simulink model "BCM_C1A_CombiSwitch_9"  (R2018b)
settings: Solver=FixedStepDiscrete  StartTime=0.0  StopTime=10.0  FixedStep=0.01  RelTol=1e-3
undefined symbols (not defined in the file or in its folder): TYP_CSW_INT_POSITION, TYP_EXT_LIGHTS, TYP_FRONT_WIPER, TYP_LIGHTING_CSW, TYP_REAR_WIPER, TYP_VEHICLE_STATE
libraries: Renault_Library x80, library_BCM x2
(part 1 of 3)
settings Model: Creator=a205328  LastModifiedBy=40005501
settings DataIOCC: LimitDataPoints=on  SaveFormat=StructureWithTime  SignalLoggingSaveFormat=ModelDataLogs
settings OptimizationCC: ExpressionDepthLimit=2147483647  LifeSpan=inf
settings DebuggingCC: UnderspecifiedInitializationDetection=Classic  MergeDetectMultiDrivingBlocksExec=none  SolverPrmCheckMsg=warning  InheritedTsInSrcMsg=none  FcnCallInpInsideContextMsg=warning  StateNameClashWarn=warning  SFUnexpectedBacktrackingDiag=warning  SFNoUnconditionalDefaultTransitionDiag=warning  SFExecutionAtInitializationDiag=none
settings HardwareCC: ProdBitPerPointer=32  ProdBitPerSizeT=32  ProdBitPerPtrDiffT=32  ProdLargestAtomicFloat=None  ProdIntDivRoundTo=Undefined  ProdEndianess=Unspecified  ProdWordSize=32  ProdHWDeviceType=32-bit Generic  TargetBitPerPointer=64  TargetBitPerSizeT=64  TargetBitPerPtrDiffT=64  TargetLongLongMode=on  TargetIntDivRoundTo=Zero  TargetEndianess=LittleEndian  TargetWordSize=64  TargetHWDeviceType=MATLAB Host  ProdEqTarget=off
settings ModelReferenceCC: PropagateSignalLabelsOutOfModel=off
settings SFSimCC: SimUseLocalCustomCode=off
settings RTWCC: Description=Generic Real-Time Target  RTWUseLocalCustomCode=off
settings CodeAppCC: StateflowObjectComments=on
settings GRTTargetCC: TargetLangStandard=C89/C90 (ANSI)  GeneratePreprocessorConditionals=Disable all  CombineOutputUpdateFcns=off  MatFileLogging=off  SupportNonFinite=off  GRTInterface=on
settings ConfigComp: CovMetricSettings=dcmw  CovHTMLOptions=-sRT=1 -aTS=1 -bRG=1 -bTC=1 -hTR=0 -nFC=0 -scm=1 -bcm=1 -xEv=0  CovHtmlReporting=on  CovSaveCumulativeToWorkspaceVar=on  CovSaveSingleToWorkspaceVar=on  CovExternalEMLEnable=off  DVMaxTestCaseSteps=500  DVTestSuiteOptimization=CombinedObjectives (Nonlinear Extended)  DVDetectDeadLogic=on  DVDetectActiveLogic=on  DVDetectDivisionByZero=off  DVDetectIntegerOverflow=off  DVSaveReport=on

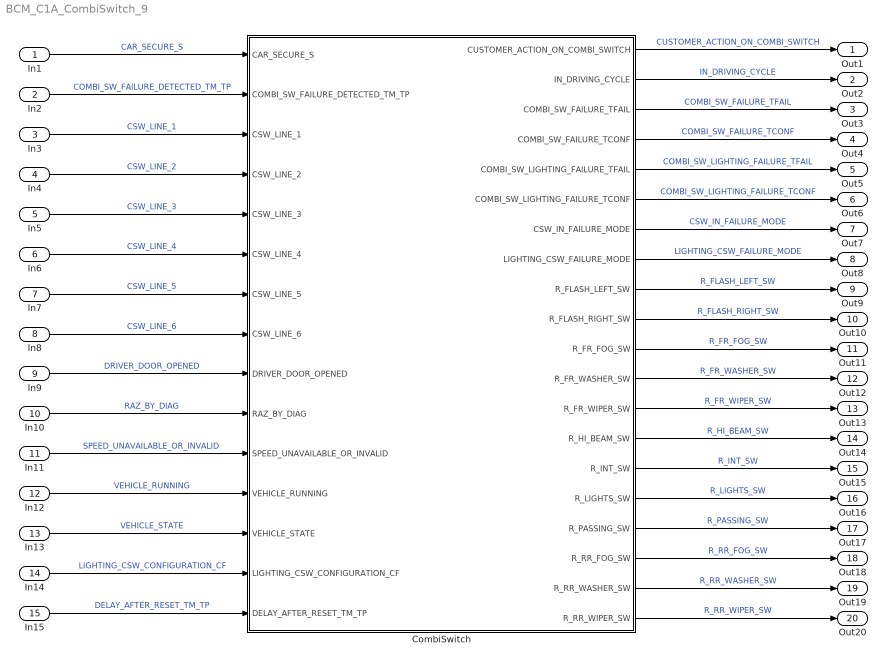
== system BCM_C1A_CombiSwitch_9 ==
  In1 : Inport
  In2 : Inport  Port=2
  In3 : Inport  Port=3
  In4 : Inport  Port=4
  In5 : Inport  Port=5
  In6 : Inport  Port=6
  In7 : Inport  Port=7
  In8 : Inport  Port=8
  In9 : Inport  Port=9
  In10 : Inport  Port=10
  In11 : Inport  Port=11
  In12 : Inport  Port=12
  In13 : Inport  Port=13
  In14 : Inport  Port=14
  In15 : Inport  Port=15
  CombiSwitch : Subsystem  Tag=[RUNNABLE]
  Out1 : Outport
  Out2 : Outport  Port=2
  Out3 : Outport  Port=3
  Out4 : Outport  Port=4
  Out5 : Outport  Port=5
  Out6 : Outport  Port=6
  Out7 : Outport  Port=7
  Out8 : Outport  Port=8
  Out9 : Outport  Port=9
  Out10 : Outport  Port=10
  Out11 : Outport  Port=11
  Out12 : Outport  Port=12
  Out13 : Outport  Port=13
  Out14 : Outport  Port=14
  Out15 : Outport  Port=15
  Out16 : Outport  Port=16
  Out17 : Outport  Port=17
  Out18 : Outport  Port=18
  Out19 : Outport  Port=19
  Out20 : Outport  Port=20
  wires:
  In1/1 -> CombiSwitch/1(CAR_SECURE_S)  "CAR_SECURE_S"
  In2/1 -> CombiSwitch/2(COMBI_SW_FAILURE_DETECTED_TM_TP)  "COMBI_SW_FAILURE_DETECTED_TM_TP"
  In3/1 -> CombiSwitch/3(CSW_LINE_1)  "CSW_LINE_1"
  In4/1 -> CombiSwitch/4(CSW_LINE_2)  "CSW_LINE_2"
  In5/1 -> CombiSwitch/5(CSW_LINE_3)  "CSW_LINE_3"
  In6/1 -> CombiSwitch/6(CSW_LINE_4)  "CSW_LINE_4"
  In7/1 -> CombiSwitch/7(CSW_LINE_5)  "CSW_LINE_5"
  In8/1 -> CombiSwitch/8(CSW_LINE_6)  "CSW_LINE_6"
  In9/1 -> CombiSwitch/9(DRIVER_DOOR_OPENED)  "DRIVER_DOOR_OPENED"
  In10/1 -> CombiSwitch/10(RAZ_BY_DIAG)  "RAZ_BY_DIAG"
  In11/1 -> CombiSwitch/11(SPEED_UNAVAILABLE_OR_INVALID)  "SPEED_UNAVAILABLE_OR_INVALID"
  In12/1 -> CombiSwitch/12(VEHICLE_RUNNING)  "VEHICLE_RUNNING"
  In13/1 -> CombiSwitch/13(VEHICLE_STATE)  "VEHICLE_STATE"
  In14/1 -> CombiSwitch/14(LIGHTING_CSW_CONFIGURATION_CF)  "LIGHTING_CSW_CONFIGURATION_CF"
  In15/1 -> CombiSwitch/15(DELAY_AFTER_RESET_TM_TP)  "DELAY_AFTER_RESET_TM_TP"
  CombiSwitch/1(CUSTOMER_ACTION_ON_COMBI_SWITCH) -> Out1/1  "CUSTOMER_ACTION_ON_COMBI_SWITCH"
  CombiSwitch/2(IN_DRIVING_CYCLE) -> Out2/1  "IN_DRIVING_CYCLE"
  CombiSwitch/3(COMBI_SW_FAILURE_TFAIL) -> Out3/1  "COMBI_SW_FAILURE_TFAIL"
  CombiSwitch/4(COMBI_SW_FAILURE_TCONF) -> Out4/1  "COMBI_SW_FAILURE_TCONF"
  CombiSwitch/5(COMBI_SW_LIGHTING_FAILURE_TFAIL) -> Out5/1  "COMBI_SW_LIGHTING_FAILURE_TFAIL"
  CombiSwitch/6(COMBI_SW_LIGHTING_FAILURE_TCONF) -> Out6/1  "COMBI_SW_LIGHTING_FAILURE_TCONF"
  CombiSwitch/7(CSW_IN_FAILURE_MODE) -> Out7/1  "CSW_IN_FAILURE_MODE"
  CombiSwitch/8(LIGHTING_CSW_FAILURE_MODE) -> Out8/1  "LIGHTING_CSW_FAILURE_MODE"
  CombiSwitch/9(R_FLASH_LEFT_SW) -> Out9/1  "R_FLASH_LEFT_SW"
  CombiSwitch/10(R_FLASH_RIGHT_SW) -> Out10/1  "R_FLASH_RIGHT_SW"
  CombiSwitch/11(R_FR_FOG_SW) -> Out11/1  "R_FR_FOG_SW"
  CombiSwitch/12(R_FR_WASHER_SW) -> Out12/1  "R_FR_WASHER_SW"
  CombiSwitch/13(R_FR_WIPER_SW) -> Out13/1  "R_FR_WIPER_SW"
  CombiSwitch/14(R_HI_BEAM_SW) -> Out14/1  "R_HI_BEAM_SW"
  CombiSwitch/15(R_INT_SW) -> Out15/1  "R_INT_SW"
  CombiSwitch/16(R_LIGHTS_SW) -> Out16/1  "R_LIGHTS_SW"
  CombiSwitch/17(R_PASSING_SW) -> Out17/1  "R_PASSING_SW"
  CombiSwitch/18(R_RR_FOG_SW) -> Out18/1  "R_RR_FOG_SW"
  CombiSwitch/19(R_RR_WASHER_SW) -> Out19/1  "R_RR_WASHER_SW"
  CombiSwitch/20(R_RR_WIPER_SW) -> Out20/1  "R_RR_WIPER_SW"

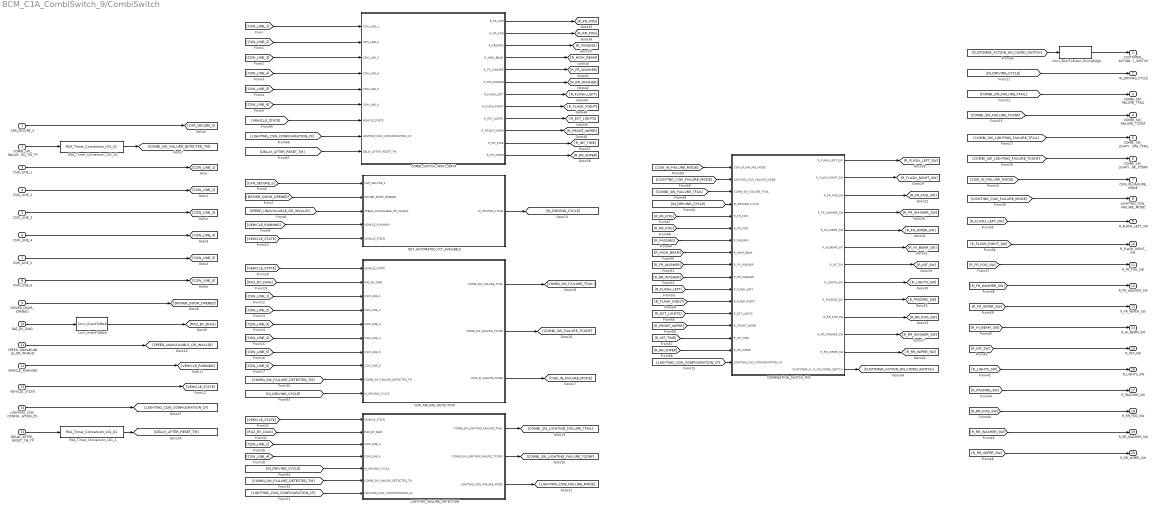
== system BCM_C1A_CombiSwitch_9/CombiSwitch ==
  CAR_SECURE_S : Inport  OutDataTypeStr=boolean
      settings: AttributesFormatString=Type : %<OutDataTypeStr>
  COMBI_SW_FAILURE_DETECTED_TM_TP : Inport  Port=2  OutDataTypeStr=uint16
      settings: AttributesFormatString=Type : %<OutDataTypeStr>
  CSW_LINE_1 : Inport  Port=3  OutDataTypeStr=boolean  PortDimensions=6
      settings: AttributesFormatString=Type : %<OutDataTypeStr>
  CSW_LINE_2 : Inport  Port=4  OutDataTypeStr=boolean  PortDimensions=6
      settings: AttributesFormatString=Type : %<OutDataTypeStr>
  CSW_LINE_3 : Inport  Port=5  OutDataTypeStr=boolean  PortDimensions=6
      settings: AttributesFormatString=Type : %<OutDataTypeStr>
  CSW_LINE_4 : Inport  Port=6  OutDataTypeStr=boolean  PortDimensions=6
      settings: AttributesFormatString=Type : %<OutDataTypeStr>
  CSW_LINE_5 : Inport  Port=7  OutDataTypeStr=boolean  PortDimensions=6
      settings: AttributesFormatString=Type : %<OutDataTypeStr>
  CSW_LINE_6 : Inport  Port=8  OutDataTypeStr=boolean  PortDimensions=6
      settings: AttributesFormatString=Type : %<OutDataTypeStr>
  DRIVER_DOOR_OPENED : Inport  Port=9  OutDataTypeStr=boolean
      settings: AttributesFormatString=Type : %<OutDataTypeStr>
  RAZ_BY_DIAG : Inport  Port=10  OutDataTypeStr=Enum: TYP_EVENT
      settings: AttributesFormatString=Type : %<OutDataTypeStr>
  SPEED_UNAVAILABLE_OR_INVALID : Inport  Port=11  OutDataTypeStr=boolean
      settings: AttributesFormatString=Type : %<OutDataTypeStr>
  VEHICLE_RUNNING : Inport  Port=12  OutDataTypeStr=boolean
      settings: AttributesFormatString=Type : %<OutDataTypeStr>
  VEHICLE_STATE : Inport  Port=13  OutDataTypeStr=Enum: TYP_VEHICLE_STATE
      settings: AttributesFormatString=Type : %<OutDataTypeStr>
  LIGHTING_CSW_CONFIGURATION_CF : Inport  Port=14  OutDataTypeStr=Enum: TYP_LIGHTING_CSW
      settings: AttributesFormatString=Type : %<OutDataTypeStr>
  DELAY_AFTER_RESET_TM_TP : Inport  Port=15  OutDataTypeStr=uint8
      settings: AttributesFormatString=Type : %<OutDataTypeStr>
  COMBINATION_SWITCH_FNS : Subsystem  Description=RQT_BCM_CSV_1_1
  COMBI_SWITCH_INPUT_DATA : Subsystem  Description=|
      | RQT_BCM_CSV_0_9
      | RQT_BCM_CSV_1_0
  CSW_FAILURE_DETECTION : Subsystem  Description=|
      | RQT_BCM_CSV_1_1  
      | RQT_BCM_CSV_1_2  
      | RQT_BCM_CSV_1_3  
      | RQT_BCM_CSV_1_3_2
  Conv_BoolToEvent_RisingEdge : library_BCM/Modeling/Conv_BoolToEvent_RisingEdge
  Conv_EventToBool : library_BCM/Modeling/Conv_EventToBool
  DET_AUTOMATED_FCT_AVAILABLE : Subsystem  Description=RQT_EXTLIGHTS_BCM_10
  LIGHTING_FAILURE_DETECTION : Subsystem  Description=|
      | RQT_BCM_CSV_1_4
      | RQT_BCM_CSV_1_7
      | RQT_BCM_CSV_1_9
  RSA_Timer_Conversion_v01_01 : Renault_Library/Complex blocks/Timers & Counters/RSA_Timer_Conversion_v01_01  Tag=[LIB]  SAMPLE_TIME_CST=CSW_SAMPLE_TIME_CST
      settings: AttributesFormatString=%<MaskType> : Ver : 01.01
  RSA_Timer_Conversion_v01_1 : Renault_Library/Complex blocks/Timers & Counters/RSA_Timer_Conversion_v01_01  Tag=[LIB]  SAMPLE_TIME_CST=CSW_SAMPLE_TIME_CST
      settings: AttributesFormatString=%<MaskType> : Ver : 01.01
  CUSTOMER_ACTION_ON_COMBI_SWITCH : Outport  OutDataTypeStr=Enum: TYP_EVENT
      settings: AttributesFormatString=Type : %<OutDataTypeStr>\nInit :%<InitialOutput>
  IN_DRIVING_CYCLE : Outport  Port=2  OutDataTypeStr=boolean
      settings: AttributesFormatString=Type : %<OutDataTypeStr>\nInit :%<InitialOutput>
  COMBI_SW_FAILURE_TFAIL : Outport  Port=3  OutDataTypeStr=boolean
      settings: AttributesFormatString=Type : %<OutDataTypeStr>\nInit :%<InitialOutput>
  COMBI_SW_FAILURE_TCONF : Outport  Port=4  OutDataTypeStr=boolean
      settings: AttributesFormatString=Type : %<OutDataTypeStr>\nInit :%<InitialOutput>
  COMBI_SW_LIGHTING_FAILURE_TFAIL : Outport  Port=5  OutDataTypeStr=boolean
      settings: AttributesFormatString=Type : %<OutDataTypeStr>\nInit :%<InitialOutput>
  COMBI_SW_LIGHTING_FAILURE_TCONF : Outport  Port=6  OutDataTypeStr=boolean
      settings: AttributesFormatString=Type : %<OutDataTypeStr>\nInit :%<InitialOutput>
  CSW_IN_FAILURE_MODE : Outport  Port=7  OutDataTypeStr=boolean
      settings: AttributesFormatString=Type : %<OutDataTypeStr>\nInit :%<InitialOutput>
  LIGHTING_CSW_FAILURE_MODE : Outport  Port=8  OutDataTypeStr=boolean
      settings: AttributesFormatString=Type : %<OutDataTypeStr>\nInit :%<InitialOutput>
  R_FLASH_LEFT_SW : Outport  Port=9  OutDataTypeStr=boolean
      settings: AttributesFormatString=Type : %<OutDataTypeStr>\nInit :%<InitialOutput>
  R_FLASH_RIGHT_SW : Outport  Port=10  OutDataTypeStr=boolean
      settings: AttributesFormatString=Type : %<OutDataTypeStr>\nInit :%<InitialOutput>
  R_FR_FOG_SW : Outport  Port=11  OutDataTypeStr=boolean
      settings: AttributesFormatString=Type : %<OutDataTypeStr>\nInit :%<InitialOutput>
  R_FR_WASHER_SW : Outport  Port=12  OutDataTypeStr=boolean
      settings: AttributesFormatString=Type : %<OutDataTypeStr>\nInit :%<InitialOutput>
  R_FR_WIPER_SW : Outport  Port=13  OutDataTypeStr=Enum: TYP_FRONT_WIPER
      settings: AttributesFormatString=Type : %<OutDataTypeStr>\nInit :%<InitialOutput>
  R_HI_BEAM_SW : Outport  Port=14  OutDataTypeStr=boolean
      settings: AttributesFormatString=Type : %<OutDataTypeStr>\nInit :%<InitialOutput>
  R_INT_SW : Outport  Port=15  OutDataTypeStr=Enum: TYP_CSW_INT_POSITION
      settings: AttributesFormatString=Type : %<OutDataTypeStr>\nInit :%<InitialOutput>
  R_LIGHTS_SW : Outport  Port=16  OutDataTypeStr=Enum: TYP_EXT_LIGHTS
      settings: AttributesFormatString=Type : %<OutDataTypeStr>\nInit :%<InitialOutput>
  R_PASSING_SW : Outport  Port=17  OutDataTypeStr=boolean
      settings: AttributesFormatString=Type : %<OutDataTypeStr>\nInit :%<InitialOutput>
  R_RR_FOG_SW : Outport  Port=18  OutDataTypeStr=boolean
      settings: AttributesFormatString=Type : %<OutDataTypeStr>\nInit :%<InitialOutput>
  R_RR_WASHER_SW : Outport  Port=19  OutDataTypeStr=boolean
      settings: AttributesFormatString=Type : %<OutDataTypeStr>\nInit :%<InitialOutput>
  R_RR_WIPER_SW : Outport  Port=20  OutDataTypeStr=Enum: TYP_REAR_WIPER
      settings: AttributesFormatString=Type : %<OutDataTypeStr>\nInit :%<InitialOutput>
  wires:
  Conv_EventToBool/1 -> [RAZ_BY_DIAG]
  [VEHICLE_STATE] -> COMBI_SWITCH_INPUT_DATA/7(VEHICLE_STATE)
  [IN_DRIVING_CYCLE] -> CSW_FAILURE_DETECTION/10(IN_DRIVING_CYCLE)
  [IN_DRIVING_CYCLE] -> LIGHTING_FAILURE_DETECTION/5(IN_DRIVING_CYCLE)
  [R_RR_WIPER] -> COMBINATION_SWITCH_FNS/16(R_RR_WIPER)
  [R_INT_TIME] -> COMBINATION_SWITCH_FNS/15(R_INT_TIME)
  [R_FRONT_WIPER] -> COMBINATION_SWITCH_FNS/14(R_FRONT_WIPER)
  [IN_DRIVING_CYCLE] -> COMBINATION_SWITCH_FNS/4(IN_DRIVING_CYCLE)
  [COMBI_SW_FAILURE_TFAIL] -> COMBINATION_SWITCH_FNS/3(COMBI_SW_FAILURE_TFAIL)
  [CSW_IN_FAILURE_MODE] -> COMBINATION_SWITCH_FNS/1(CSW_IN_FAILURE_MODE)
  [LIGHTING_CSW_FAILURE_MODE] -> COMBINATION_SWITCH_FNS/2(LIGHTING_CSW_FAILURE_MODE)
  [R_EXT_LIGHTS] -> COMBINATION_SWITCH_FNS/13(R_EXT_LIGHTS)
  [R_FLASH_RIGHT] -> COMBINATION_SWITCH_FNS/12(R_FLASH_RIGHT)
  [R_FLASH_LEFT] -> COMBINATION_SWITCH_FNS/11(R_FLASH_LEFT)
  [R_RR_WASHER] -> COMBINATION_SWITCH_FNS/10(R_RR_WASHER)
  [R_FR_WASHER] -> COMBINATION_SWITCH_FNS/9(R_FR_WASHER)
  [R_HIGH_BEAM] -> COMBINATION_SWITCH_FNS/8(R_HIGH_BEAM)
  [R_PASSING] -> COMBINATION_SWITCH_FNS/7(R_PASSING)
  [R_RR_FOG] -> COMBINATION_SWITCH_FNS/6(R_RR_FOG)
  [R_FR_FOG] -> COMBINATION_SWITCH_FNS/5(R_FR_FOG)
  COMBI_SWITCH_INPUT_DATA/12(R_RR_WIPER) -> [R_RR_WIPER]
  COMBI_SWITCH_INPUT_DATA/11(R_INT_TIME) -> [R_INT_TIME]
  COMBI_SWITCH_INPUT_DATA/10(R_FRONT_WIPER) -> [R_FRONT_WIPER]
  COMBI_SWITCH_INPUT_DATA/9(R_EXT_LIGHTS) -> [R_EXT_LIGHTS]
  COMBI_SWITCH_INPUT_DATA/8(R_FLASH_RIGHT) -> [R_FLASH_RIGHT]
  COMBI_SWITCH_INPUT_DATA/7(R_FLASH_LEFT) -> [R_FLASH_LEFT]
  COMBI_SWITCH_INPUT_DATA/6(R_RR_WASHER) -> [R_RR_WASHER]
  COMBI_SWITCH_INPUT_DATA/5(R_FR_WASHER) -> [R_FR_WASHER]
  COMBI_SWITCH_INPUT_DATA/4(R_HIGH_BEAM) -> [R_HIGH_BEAM]
  COMBI_SWITCH_INPUT_DATA/3(R_PASSING) -> [R_PASSING]
  COMBI_SWITCH_INPUT_DATA/2(R_RR_FOG) -> [R_RR_FOG]
  COMBI_SWITCH_INPUT_DATA/1(R_FR_FOG) -> [R_FR_FOG]
  COMBINATION_SWITCH_FNS/5(R_FR_WIPER_SW) -> [R_FR_WIPER_SW]
  COMBINATION_SWITCH_FNS/10(R_RR_FOG_SW) -> [R_RR_FOG_SW]
  COMBINATION_SWITCH_FNS/3(R_FR_FOG_SW) -> [R_FR_FOG_SW]
  COMBINATION_SWITCH_FNS/4(R_FR_WASHER_SW) -> [R_FR_WASHER_SW]
  COMBINATION_SWITCH_FNS/9(R_PASSING_SW) -> [R_PASSING_SW]
  COMBINATION_SWITCH_FNS/11(R_RR_WASHER_SW) -> [R_RR_WASHER_SW]
  COMBINATION_SWITCH_FNS/2(R_FLASH_RIGHT_SW) -> [R_FLASH_RIGHT_SW]
  COMBINATION_SWITCH_FNS/1(R_FLASH_LEFT_SW) -> [R_FLASH_LEFT_SW]
  COMBINATION_SWITCH_FNS/7(R_INT_SW) -> [R_INT_SW]
  COMBINATION_SWITCH_FNS/12(R_RR_WIPER_SW) -> [R_RR_WIPER_SW]
  COMBINATION_SWITCH_FNS/13(CUSTOMER_ACTION_ON_COMBI_SWITCH) -> [CUSTOMER_ACTION_ON_COMBI_SWITCH]
  COMBINATION_SWITCH_FNS/6(R_HI_BEAM_SW) -> [R_HI_BEAM_SW]
  COMBINATION_SWITCH_FNS/8(R_LIGHTS_SW) -> [R_LIGHTS_SW]
  LIGHTING_FAILURE_DETECTION/3(LIGHTING_CSW_FAILURE_MODE) -> [LIGHTING_CSW_FAILURE_MODE]
  LIGHTING_FAILURE_DETECTION/2(COMBI_SW_LIGHTING_FAILURE_TCONF) -> [COMBI_SW_LIGHTING_FAILURE_TCONF]
  LIGHTING_FAILURE_DETECTION/1(COMBI_SW_LIGHTING_FAILURE_TFAIL) -> [COMBI_SW_LIGHTING_FAILURE_TFAIL]
  [COMBI_SW_FAILURE_DETECTED_TM] -> LIGHTING_FAILURE_DETECTION/6(COMBI_SW_FAILURE_DETECTED_TM)
  [CSW_LINE_4] -> LIGHTING_FAILURE_DETECTION/4(CSW_LINE_4)
  [CSW_LINE_2] -> LIGHTING_FAILURE_DETECTION/3(CSW_LINE_2)
  [RAZ_BY_DIAG] -> LIGHTING_FAILURE_DETECTION/2(RAZ_BY_DIAG)
  [VEHICLE_STATE] -> LIGHTING_FAILURE_DETECTION/1(VEHICLE_STATE)
  [COMBI_SW_FAILURE_DETECTED_TM] -> CSW_FAILURE_DETECTION/9(COMBI_SW_FAILURE_DETECTED_TM)
  [CSW_LINE_6] -> CSW_FAILURE_DETECTION/8(CSW_LINE_6)
  [CSW_LINE_5] -> CSW_FAILURE_DETECTION/7(CSW_LINE_5)
  [CSW_LINE_4] -> CSW_FAILURE_DETECTION/6(CSW_LINE_4)
  [CSW_LINE_3] -> CSW_FAILURE_DETECTION/5(CSW_LINE_3)
  [CSW_LINE_2] -> CSW_FAILURE_DETECTION/4(CSW_LINE_2)
  [CSW_LINE_1] -> CSW_FAILURE_DETECTION/3(CSW_LINE_1)
  [RAZ_BY_DIAG] -> CSW_FAILURE_DETECTION/2(RAZ_BY_DIAG)
  [VEHICLE_STATE] -> CSW_FAILURE_DETECTION/1(VEHICLE_STATE)
  CSW_LINE_6/1 -> [CSW_LINE_6]
  CSW_LINE_5/1 -> [CSW_LINE_5]
  CSW_LINE_4/1 -> [CSW_LINE_4]
  CSW_LINE_3/1 -> [CSW_LINE_3]
  CSW_LINE_2/1 -> [CSW_LINE_2]
  CSW_LINE_1/1 -> [CSW_LINE_1]
  DET_AUTOMATED_FCT_AVAILABLE/1(IN_DRIVING_CYCLE) -> [IN_DRIVING_CYCLE]
  [VEHICLE_STATE] -> DET_AUTOMATED_FCT_AVAILABLE/5(VEHICLE_STATE)
  [VEHICLE_RUNNING] -> DET_AUTOMATED_FCT_AVAILABLE/4(VEHICLE_RUNNING)
  [SPEED_UNAVAILABLE_OR_INVALID] -> DET_AUTOMATED_FCT_AVAILABLE/3(SPEED_UNAVAILABLE_OR_INVALID)
  [DRIVER_DOOR_OPENED] -> DET_AUTOMATED_FCT_AVAILABLE/2(DRIVER_DOOR_OPENED)
  [CAR_SECURE_S] -> DET_AUTOMATED_FCT_AVAILABLE/1(CAR_SECURE_S)
  DRIVER_DOOR_OPENED/1 -> [DRIVER_DOOR_OPENED]
  RAZ_BY_DIAG/1 -> Conv_EventToBool/1
  SPEED_UNAVAILABLE_OR_INVALID/1 -> [SPEED_UNAVAILABLE_OR_INVALID]
  VEHICLE_RUNNING/1 -> [VEHICLE_RUNNING]
  VEHICLE_STATE/1 -> [VEHICLE_STATE]
  COMBI_SW_FAILURE_DETECTED_TM_TP/1 -> RSA_Timer_Conversion_v01_01/1
  CAR_SECURE_S/1 -> [CAR_SECURE_S]
  [CSW_LINE_6] -> COMBI_SWITCH_INPUT_DATA/6(CSW_LINE_6)
  [CSW_LINE_5] -> COMBI_SWITCH_INPUT_DATA/5(CSW_LINE_5)
  [CSW_LINE_4] -> COMBI_SWITCH_INPUT_DATA/4(CSW_LINE_4)
  [CSW_LINE_3] -> COMBI_SWITCH_INPUT_DATA/3(CSW_LINE_3)
  [CSW_LINE_2] -> COMBI_SWITCH_INPUT_DATA/2(CSW_LINE_2)
  [CSW_LINE_1] -> COMBI_SWITCH_INPUT_DATA/1(CSW_LINE_1)
  LIGHTING_CSW_CONFIGURATION_CF/1 -> [LIGHTING_CSW_CONFIGURATION_CF]
  [LIGHTING_CSW_CONFIGURATION_CF] -> COMBI_SWITCH_INPUT_DATA/8(LIGHTING_CSW_CONFIGURATION_CF)
  RSA_Timer_Conversion_v01_01/1 -> [COMBI_SW_FAILURE_DETECTED_TM]
  [LIGHTING_CSW_CONFIGURATION_CF] -> LIGHTING_FAILURE_DETECTION/7(LIGHTING_CSW_CONFIGURATION_CF)
  [LIGHTING_CSW_CONFIGURATION_CF] -> COMBINATION_SWITCH_FNS/17(LIGHTING_CSW_CONFIGURATION_CF)
  DELAY_AFTER_RESET_TM_TP/1 -> RSA_Timer_Conversion_v01_1/1
  RSA_Timer_Conversion_v01_1/1 -> [DELAY_AFTER_RESET_TM]
  [DELAY_AFTER_RESET_TM] -> COMBI_SWITCH_INPUT_DATA/9(DELAY_AFTER_RESET_TM)
  CSW_FAILURE_DETECTION/2(COMBI_SW_FAILURE_TCONF) -> [COMBI_SW_FAILURE_TCONF]
  CSW_FAILURE_DETECTION/3(CSW_IN_FAILURE_MODE) -> [CSW_IN_FAILURE_MODE]
  CSW_FAILURE_DETECTION/1(COMBI_SW_FAILURE_TFAIL) -> [COMBI_SW_FAILURE_TFAIL]
  [COMBI_SW_FAILURE_TFAIL] -> COMBI_SW_FAILURE_TFAIL/1
  [COMBI_SW_FAILURE_TCONF] -> COMBI_SW_FAILURE_TCONF/1
  [IN_DRIVING_CYCLE] -> IN_DRIVING_CYCLE/1
  [CSW_IN_FAILURE_MODE] -> CSW_IN_FAILURE_MODE/1
  [COMBI_SW_LIGHTING_FAILURE_TCONF] -> COMBI_SW_LIGHTING_FAILURE_TCONF/1
  [COMBI_SW_LIGHTING_FAILURE_TFAIL] -> COMBI_SW_LIGHTING_FAILURE_TFAIL/1
  [LIGHTING_CSW_FAILURE_MODE] -> LIGHTING_CSW_FAILURE_MODE/1
  [CUSTOMER_ACTION_ON_COMBI_SWITCH] -> Conv_BoolToEvent_RisingEdge/1
  [R_FLASH_LEFT_SW] -> R_FLASH_LEFT_SW/1
  [R_FLASH_RIGHT_SW] -> R_FLASH_RIGHT_SW/1
  [R_FR_FOG_SW] -> R_FR_FOG_SW/1
  [R_FR_WASHER_SW] -> R_FR_WASHER_SW/1
  [R_FR_WIPER_SW] -> R_FR_WIPER_SW/1
  [R_HI_BEAM_SW] -> R_HI_BEAM_SW/1
  [R_INT_SW] -> R_INT_SW/1
  [R_LIGHTS_SW] -> R_LIGHTS_SW/1
  [R_PASSING_SW] -> R_PASSING_SW/1
  [R_RR_FOG_SW] -> R_RR_FOG_SW/1
  [R_RR_WASHER_SW] -> R_RR_WASHER_SW/1
  [R_RR_WIPER_SW] -> R_RR_WIPER_SW/1
  Conv_BoolToEvent_RisingEdge/1 -> CUSTOMER_ACTION_ON_COMBI_SWITCH/1

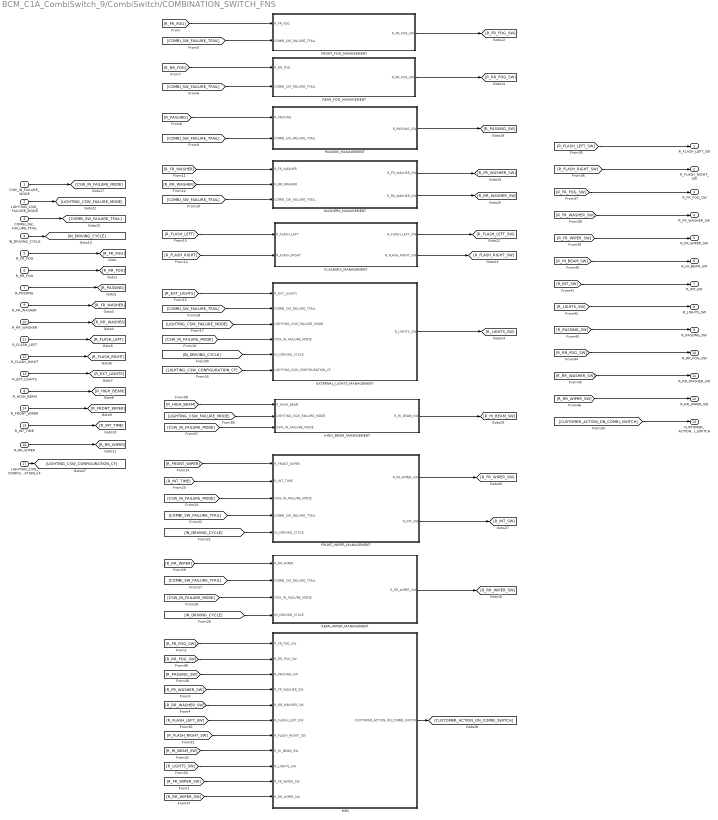
== system BCM_C1A_CombiSwitch_9/CombiSwitch/COMBINATION_SWITCH_FNS ==
  CSW_IN_FAILURE_MODE : Inport  OutDataTypeStr=boolean
      settings: AttributesFormatString=Type : %<OutDataTypeStr>
  LIGHTING_CSW_FAILURE_MODE : Inport  Port=2  OutDataTypeStr=boolean
      settings: AttributesFormatString=Type : %<OutDataTypeStr>
  COMBI_SW_FAILURE_TFAIL : Inport  Port=3  OutDataTypeStr=boolean
      settings: AttributesFormatString=Type : %<OutDataTypeStr>
  IN_DRIVING_CYCLE : Inport  Port=4  OutDataTypeStr=boolean
      settings: AttributesFormatString=Type : %<OutDataTypeStr>
  R_FR_FOG : Inport  Port=5  OutDataTypeStr=boolean
      settings: AttributesFormatString=Type : %<OutDataTypeStr>
  R_RR_FOG : Inport  Port=6  OutDataTypeStr=boolean
      settings: AttributesFormatString=Type : %<OutDataTypeStr>
  R_PASSING : Inport  Port=7  OutDataTypeStr=boolean
      settings: AttributesFormatString=Type : %<OutDataTypeStr>
  R_HIGH_BEAM : Inport  Port=8  OutDataTypeStr=boolean
      settings: AttributesFormatString=Type : %<OutDataTypeStr>
  R_FR_WASHER : Inport  Port=9  OutDataTypeStr=boolean
      settings: AttributesFormatString=Type : %<OutDataTypeStr>
  R_RR_WASHER : Inport  Port=10  OutDataTypeStr=boolean
      settings: AttributesFormatString=Type : %<OutDataTypeStr>
  R_FLASH_LEFT : Inport  Port=11  OutDataTypeStr=boolean
      settings: AttributesFormatString=Type : %<OutDataTypeStr>
  R_FLASH_RIGHT : Inport  Port=12  OutDataTypeStr=boolean
      settings: AttributesFormatString=Type : %<OutDataTypeStr>
  R_EXT_LIGHTS : Inport  Port=13  OutDataTypeStr=Enum: TYP_EXT_LIGHTS
      settings: AttributesFormatString=Type : %<OutDataTypeStr>
  R_FRONT_WIPER : Inport  Port=14  OutDataTypeStr=Enum: TYP_FRONT_WIPER
      settings: AttributesFormatString=Type : %<OutDataTypeStr>
  R_INT_TIME : Inport  Port=15  OutDataTypeStr=Enum: TYP_CSW_INT_POSITION
      settings: AttributesFormatString=Type : %<OutDataTypeStr>
  R_RR_WIPER : Inport  Port=16  OutDataTypeStr=Enum: TYP_REAR_WIPER
      settings: AttributesFormatString=Type : %<OutDataTypeStr>
  LIGHTING_CSW_CONFIGURATION_CF : Inport  Port=17  OutDataTypeStr=Enum: TYP_LIGHTING_CSW
      settings: AttributesFormatString=Type : %<OutDataTypeStr>
  EXTERNAL_LIGHTS_MANAGEMENT : Subsystem  Description=|
      | RQT_BCM_CSV_1_4
      | RQT_BCM_CSV_2_1
      | RQT_BCM_CSV_2_2
      | RQT_BCM_CSV_2_5
      | RQT_BCM_CSV_2_6
      | RQT_BCM_CSV_2_7
  FLASHERS_MANAGEMENT : Subsystem  Description=|
      | RQT_BCM_CSV_2_0
      | RQT_BCM_CSV_2_1
  FRONT_FOG_MANAGEMENT : Subsystem  Description=RQT_BCM_CSV_2_3
  FRONT_WIPER_MANAGEMENT : Subsystem  Description=|
      | RQT_BCM_CSV_3_1
      | RQT_BCM_CSV_3_2
      | RQT_BCM_CSV_3_3
      | RQT_BCM_CSV_3_4
  HIGH_BEAM_MANAGEMENT : Subsystem  Description=|
      | RQT_BCM_CSV_1_4
      | RQT_BCM_CSV_2_6
      | RQT_BCM_CSV_2_7
      | RQT_BCM_CSV_2_8
  MMI : Subsystem  Description=RQT_HMI_PCFN_BCM.01
  PASSING_MANAGEMENT : Subsystem  Description=|
      | RQT_BCM_CSV_2_1
      | RQT_BCM_CSV_2_2
  REAR_FOG_MANAGEMENT : Subsystem  Description=RQT_BCM_CSV_2_3
  REAR_WIPER_MANAGEMENT : Subsystem  Description=|
      | RQT_BCM_CSV_3_3
      | RQT_BCM_CSV_3_6
  WASHERS_MANAGEMENT : Subsystem  Description=RQT_BCM_CSV_3_7
  R_FLASH_LEFT_SW : Outport  OutDataTypeStr=boolean
      settings: AttributesFormatString=Type : %<OutDataTypeStr>\nInit :%<InitialOutput>
  R_FLASH_RIGHT_SW : Outport  Port=2  OutDataTypeStr=boolean
      settings: AttributesFormatString=Type : %<OutDataTypeStr>\nInit :%<InitialOutput>
  R_FR_FOG_SW : Outport  Port=3  OutDataTypeStr=boolean
      settings: AttributesFormatString=Type : %<OutDataTypeStr>\nInit :%<InitialOutput>
  R_FR_WASHER_SW : Outport  Port=4  OutDataTypeStr=boolean
      settings: AttributesFormatString=Type : %<OutDataTypeStr>\nInit :%<InitialOutput>
  R_FR_WIPER_SW : Outport  Port=5  OutDataTypeStr=Enum: TYP_FRONT_WIPER
      settings: AttributesFormatString=Type : %<OutDataTypeStr>\nInit :%<InitialOutput>
  R_HI_BEAM_SW : Outport  Port=6  OutDataTypeStr=boolean
      settings: AttributesFormatString=Type : %<OutDataTypeStr>\nInit :%<InitialOutput>
  R_INT_SW : Outport  Port=7  OutDataTypeStr=Enum: TYP_CSW_INT_POSITION
      settings: AttributesFormatString=Type : %<OutDataTypeStr>\nInit :%<InitialOutput>
  R_LIGHTS_SW : Outport  Port=8  OutDataTypeStr=Enum: TYP_EXT_LIGHTS
      settings: AttributesFormatString=Type : %<OutDataTypeStr>\nInit :%<InitialOutput>
  R_PASSING_SW : Outport  Port=9  OutDataTypeStr=boolean
      settings: AttributesFormatString=Type : %<OutDataTypeStr>\nInit :%<InitialOutput>
  R_RR_FOG_SW : Outport  Port=10  OutDataTypeStr=boolean
      settings: AttributesFormatString=Type : %<OutDataTypeStr>\nInit :%<InitialOutput>
  R_RR_WASHER_SW : Outport  Port=11  OutDataTypeStr=boolean
      settings: AttributesFormatString=Type : %<OutDataTypeStr>\nInit :%<InitialOutput>
  R_RR_WIPER_SW : Outport  Port=12  OutDataTypeStr=Enum: TYP_REAR_WIPER
      settings: AttributesFormatString=Type : %<OutDataTypeStr>\nInit :%<InitialOutput>
  CUSTOMER_ACTION_ON_COMBI_SWITCH : Outport  Port=13  OutDataTypeStr=boolean
      settings: AttributesFormatString=Type : %<OutDataTypeStr>\nInit :%<InitialOutput>
  wires:
  [IN_DRIVING_CYCLE] -> REAR_WIPER_MANAGEMENT/4(IN_DRIVING_CYCLE)
  [CSW_IN_FAILURE_MODE] -> REAR_WIPER_MANAGEMENT/3(CSW_IN_FAILURE_MODE)
  [IN_DRIVING_CYCLE] -> EXTERNAL_LIGHTS_MANAGEMENT/5(IN_DRIVING_CYCLE)
  MMI/1(CUSTOMER_ACTION_ON_COMBI_SWITCH) -> [CUSTOMER_ACTION_ON_COMBI_SWITCH]
  FRONT_WIPER_MANAGEMENT/2(R_INT_SW) -> [R_INT_SW]
  REAR_WIPER_MANAGEMENT/1(R_RR_WIPER_SW) -> [R_RR_WIPER_SW]
  FRONT_WIPER_MANAGEMENT/1(R_FR_WIPER_SW) -> [R_FR_WIPER_SW]
  EXTERNAL_LIGHTS_MANAGEMENT/1(R_LIGHTS_SW) -> [R_LIGHTS_SW]
  FLASHERS_MANAGEMENT/2(R_FLASH_RIGHT_SW) -> [R_FLASH_RIGHT_SW]
  FLASHERS_MANAGEMENT/1(R_FLASH_LEFT_SW) -> [R_FLASH_LEFT_SW]
  WASHERS_MANAGEMENT/2(R_RR_WASHER_SW) -> [R_RR_WASHER_SW]
  WASHERS_MANAGEMENT/1(R_FR_WASHER_SW) -> [R_FR_WASHER_SW]
  PASSING_MANAGEMENT/1(R_PASSING_SW) -> [R_PASSING_SW]
  REAR_FOG_MANAGEMENT/1(R_RR_FOG_SW) -> [R_RR_FOG_SW]
  FRONT_FOG_MANAGEMENT/1(R_FR_FOG_SW) -> [R_FR_FOG_SW]
  [R_RR_WIPER_SW] -> MMI/11(R_RR_WIPER_SW)
  [R_FR_WIPER_SW] -> MMI/10(R_FR_WIPER_SW)
  [R_LIGHTS_SW] -> MMI/9(R_LIGHTS_SW)
  [R_HI_BEAM_SW] -> MMI/8(R_HI_BEAM_SW)
  [R_FLASH_RIGHT_SW] -> MMI/7(R_FLASH_RIGHT_SW)
  [R_FLASH_LEFT_SW] -> MMI/6(R_FLASH_LEFT_SW)
  [R_RR_WASHER_SW] -> MMI/5(R_RR_WASHER_SW)
  [R_FR_WASHER_SW] -> MMI/4(R_FR_WASHER_SW)
  [R_PASSING_SW] -> MMI/3(R_PASSING_SW)
  [R_RR_FOG_SW] -> MMI/2(R_RR_FOG_SW)
  [R_FR_FOG_SW] -> MMI/1(R_FR_FOG_SW)
  [CUSTOMER_ACTION_ON_COMBI_SWITCH] -> CUSTOMER_ACTION_ON_COMBI_SWITCH/1
  [COMBI_SW_FAILURE_TFAIL] -> REAR_WIPER_MANAGEMENT/2(COMBI_SW_FAILURE_TFAIL)
  [R_RR_WIPER] -> REAR_WIPER_MANAGEMENT/1(R_RR_WIPER)
  R_RR_WIPER/1 -> [R_RR_WIPER]
  R_INT_TIME/1 -> [R_INT_TIME]
  R_FRONT_WIPER/1 -> [R_FRONT_WIPER]
  [IN_DRIVING_CYCLE] -> FRONT_WIPER_MANAGEMENT/5(IN_DRIVING_CYCLE)
  [COMBI_SW_FAILURE_TFAIL] -> FRONT_WIPER_MANAGEMENT/4(COMBI_SW_FAILURE_TFAIL)
  [CSW_IN_FAILURE_MODE] -> FRONT_WIPER_MANAGEMENT/3(CSW_IN_FAILURE_MODE)
  [R_INT_TIME] -> FRONT_WIPER_MANAGEMENT/2(R_INT_TIME)
  [R_FRONT_WIPER] -> FRONT_WIPER_MANAGEMENT/1(R_FRONT_WIPER)
  [CSW_IN_FAILURE_MODE] -> EXTERNAL_LIGHTS_MANAGEMENT/4(CSW_IN_FAILURE_MODE)
  [LIGHTING_CSW_FAILURE_MODE] -> EXTERNAL_LIGHTS_MANAGEMENT/3(LIGHTING_CSW_FAILURE_MODE)
  [COMBI_SW_FAILURE_TFAIL] -> EXTERNAL_LIGHTS_MANAGEMENT/2(COMBI_SW_FAILURE_TFAIL)
  [R_EXT_LIGHTS] -> EXTERNAL_LIGHTS_MANAGEMENT/1(R_EXT_LIGHTS)
  R_HIGH_BEAM/1 -> [R_HIGH_BEAM]
  R_EXT_LIGHTS/1 -> [R_EXT_LIGHTS]
  R_FLASH_LEFT/1 -> [R_FLASH_LEFT]
  R_FLASH_RIGHT/1 -> [R_FLASH_RIGHT]
  [R_FLASH_RIGHT] -> FLASHERS_MANAGEMENT/2(R_FLASH_RIGHT)
  [R_FLASH_LEFT] -> FLASHERS_MANAGEMENT/1(R_FLASH_LEFT)
  R_FR_WASHER/1 -> [R_FR_WASHER]
  R_RR_WASHER/1 -> [R_RR_WASHER]
  [R_RR_WASHER] -> WASHERS_MANAGEMENT/2(R_RR_WASHER)
  [R_FR_WASHER] -> WASHERS_MANAGEMENT/1(R_FR_WASHER)
  [COMBI_SW_FAILURE_TFAIL] -> WASHERS_MANAGEMENT/3(COMBI_SW_FAILURE_TFAIL)
  [COMBI_SW_FAILURE_TFAIL] -> PASSING_MANAGEMENT/2(COMBI_SW_FAILURE_TFAIL)
  [R_PASSING] -> PASSING_MANAGEMENT/1(R_PASSING)
  R_PASSING/1 -> [R_PASSING]
  [COMBI_SW_FAILURE_TFAIL] -> REAR_FOG_MANAGEMENT/2(COMBI_SW_FAILURE_TFAIL)
  [R_RR_FOG] -> REAR_FOG_MANAGEMENT/1(R_RR_FOG)
  R_RR_FOG/1 -> [R_RR_FOG]
  [COMBI_SW_FAILURE_TFAIL] -> FRONT_FOG_MANAGEMENT/2(COMBI_SW_FAILURE_TFAIL)
  CSW_IN_FAILURE_MODE/1 -> [CSW_IN_FAILURE_MODE]
  COMBI_SW_FAILURE_TFAIL/1 -> [COMBI_SW_FAILURE_TFAIL]
  LIGHTING_CSW_FAILURE_MODE/1 -> [LIGHTING_CSW_FAILURE_MODE]
  IN_DRIVING_CYCLE/1 -> [IN_DRIVING_CYCLE]
  [R_FR_FOG] -> FRONT_FOG_MANAGEMENT/1(R_FR_FOG)
  R_FR_FOG/1 -> [R_FR_FOG]
  [R_RR_WIPER_SW] -> R_RR_WIPER_SW/1
  [R_RR_WASHER_SW] -> R_RR_WASHER_SW/1
  [R_RR_FOG_SW] -> R_RR_FOG_SW/1
  [R_PASSING_SW] -> R_PASSING_SW/1
  [R_LIGHTS_SW] -> R_LIGHTS_SW/1
  [R_INT_SW] -> R_INT_SW/1
  [R_HI_BEAM_SW] -> R_HI_BEAM_SW/1
  [R_FR_WIPER_SW] -> R_FR_WIPER_SW/1
  [R_FR_WASHER_SW] -> R_FR_WASHER_SW/1
  [R_FR_FOG_SW] -> R_FR_FOG_SW/1
  [R_FLASH_RIGHT_SW] -> R_FLASH_RIGHT_SW/1
  [R_FLASH_LEFT_SW] -> R_FLASH_LEFT_SW/1
  HIGH_BEAM_MANAGEMENT/1(R_HI_BEAM_SW) -> [R_HI_BEAM_SW]
  [LIGHTING_CSW_FAILURE_MODE] -> HIGH_BEAM_MANAGEMENT/2(LIGHTING_CSW_FAILURE_MODE)
  [CSW_IN_FAILURE_MODE] -> HIGH_BEAM_MANAGEMENT/3(CSW_IN_FAILURE_MODE)
  [R_HIGH_BEAM] -> HIGH_BEAM_MANAGEMENT/1(R_HIGH_BEAM)
  [LIGHTING_CSW_CONFIGURATION_CF] -> EXTERNAL_LIGHTS_MANAGEMENT/6(LIGHTING_CSW_CONFIGURATION_CF)
  LIGHTING_CSW_CONFIGURATION_CF/1 -> [LIGHTING_CSW_CONFIGURATION_CF]

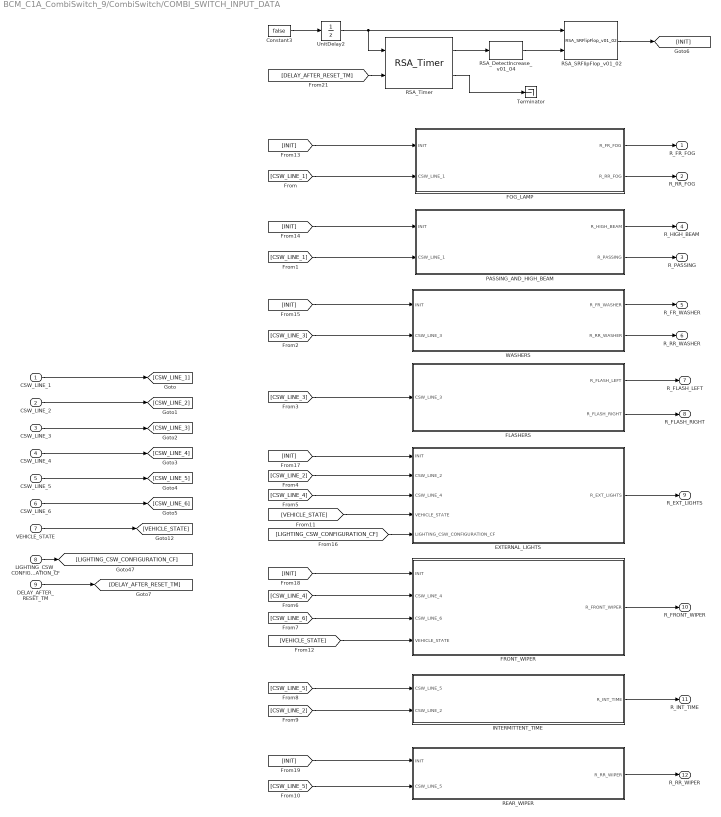
== system BCM_C1A_CombiSwitch_9/CombiSwitch/COMBI_SWITCH_INPUT_DATA ==
  CSW_LINE_1 : Inport  OutDataTypeStr=boolean  PortDimensions=6
      settings: AttributesFormatString=Type : %<OutDataTypeStr>
  CSW_LINE_2 : Inport  Port=2  OutDataTypeStr=boolean  PortDimensions=6
      settings: AttributesFormatString=Type : %<OutDataTypeStr>
  CSW_LINE_3 : Inport  Port=3  OutDataTypeStr=boolean  PortDimensions=6
      settings: AttributesFormatString=Type : %<OutDataTypeStr>
  CSW_LINE_4 : Inport  Port=4  OutDataTypeStr=boolean  PortDimensions=6
      settings: AttributesFormatString=Type : %<OutDataTypeStr>
  CSW_LINE_5 : Inport  Port=5  OutDataTypeStr=boolean  PortDimensions=6
      settings: AttributesFormatString=Type : %<OutDataTypeStr>
  CSW_LINE_6 : Inport  Port=6  OutDataTypeStr=boolean  PortDimensions=6
      settings: AttributesFormatString=Type : %<OutDataTypeStr>
  VEHICLE_STATE : Inport  Port=7  OutDataTypeStr=Enum: TYP_VEHICLE_STATE
      settings: AttributesFormatString=Type : %<OutDataTypeStr>
  LIGHTING_CSW_CONFIGURATION_CF : Inport  Port=8  OutDataTypeStr=Enum: TYP_LIGHTING_CSW
      settings: AttributesFormatString=Type : %<OutDataTypeStr>
  DELAY_AFTER_RESET_TM : Inport  Port=9  OutDataTypeStr=uint8
      settings: AttributesFormatString=Type : %<OutDataTypeStr>
  Constant3 : Constant  Value=false  OutDataTypeStr=boolean  SampleTime=-1
  EXTERNAL_LIGHTS : Subsystem  Description=RQT_BCM_CSV_1_8_2
  FLASHERS : Subsystem
  FOG_LAMP : Subsystem
  FRONT_WIPER : Subsystem  Description=RQT_BCM_CSV_1_8_2
  INTERMITTENT_TIME : Subsystem
  PASSING_AND_HIGH_BEAM : Subsystem
  REAR_WIPER : Subsystem
  RSA_DetectIncrease_v01_04 : Renault_Library/Complex blocks/Logic & Bit Operations/RSA_DetectIncrease_v01_04  Tag=[LIB]  Description=RQT_BCM_CSV_4_1  chkini=off  vinit=false
      settings: AttributesFormatString=%<MaskType> : Ver : 01.04\nCompare the Input with Initial Value = %<chkini>\nInitial Value : = %<vinit>
  RSA_SRFlipFlop_v01_02 : Renault_Library/Complex blocks/Flip-Flop/RSA_SRFlipFlop_v01_02  Tag=[LIB]  Description=RQT_BCM_CSV_4_1  IC=false
      settings: AttributesFormatString=%<MaskType> : Ver : 01.02\nInitial Condition = %<IC>
  RSA_Timer : Renault_Library/Complex blocks/Timers & Counters/RSA_Timer  Tag=[LIB]  Description=RQT_BCM_CSV_4_1  timeoutinit=CSW_ZERO_CST  initinit=CSW_ZERO_CST  st=CSW_ONE_CST
      settings: AttributesFormatString=%<MaskType> : Ver : 01.03\nTimeout output initialisation=%<timeoutinit>\nInit input initialisation=%<initinit>
  Terminator : Terminator
  UnitDelay2 : UnitDelay  InitialCondition=true  SampleTime=-1
      settings: AttributesFormatString=IC = %<X0>
  WASHERS : Subsystem
  R_FR_FOG : Outport  OutDataTypeStr=boolean
      settings: AttributesFormatString=Type : %<OutDataTypeStr>\nInit :%<InitialOutput>
  R_RR_FOG : Outport  Port=2  OutDataTypeStr=boolean
      settings: AttributesFormatString=Type : %<OutDataTypeStr>\nInit :%<InitialOutput>
  R_PASSING : Outport  Port=3  OutDataTypeStr=boolean
      settings: AttributesFormatString=Type : %<OutDataTypeStr>\nInit :%<InitialOutput>
  R_HIGH_BEAM : Outport  Port=4  OutDataTypeStr=boolean
      settings: AttributesFormatString=Type : %<OutDataTypeStr>\nInit :%<InitialOutput>
  R_FR_WASHER : Outport  Port=5  OutDataTypeStr=boolean
      settings: AttributesFormatString=Type : %<OutDataTypeStr>\nInit :%<InitialOutput>
  R_RR_WASHER : Outport  Port=6  OutDataTypeStr=boolean
      settings: AttributesFormatString=Type : %<OutDataTypeStr>\nInit :%<InitialOutput>
  R_FLASH_LEFT : Outport  Port=7  OutDataTypeStr=boolean
      settings: AttributesFormatString=Type : %<OutDataTypeStr>\nInit :%<InitialOutput>
  R_FLASH_RIGHT : Outport  Port=8  OutDataTypeStr=boolean
      settings: AttributesFormatString=Type : %<OutDataTypeStr>\nInit :%<InitialOutput>
  R_EXT_LIGHTS : Outport  Port=9  OutDataTypeStr=Enum: TYP_EXT_LIGHTS
      settings: AttributesFormatString=Type : %<OutDataTypeStr>\nInit :%<InitialOutput>
  R_FRONT_WIPER : Outport  Port=10  OutDataTypeStr=Enum: TYP_FRONT_WIPER
      settings: AttributesFormatString=Type : %<OutDataTypeStr>\nInit :%<InitialOutput>
  R_INT_TIME : Outport  Port=11  OutDataTypeStr=Enum: TYP_CSW_INT_POSITION
      settings: AttributesFormatString=Type : %<OutDataTypeStr>\nInit :%<InitialOutput>
  R_RR_WIPER : Outport  Port=12  OutDataTypeStr=Enum: TYP_REAR_WIPER
      settings: AttributesFormatString=Type : %<OutDataTypeStr>\nInit :%<InitialOutput>
  wires:
  INTERMITTENT_TIME/1(R_INT_TIME) -> R_INT_TIME/1
  [INIT] -> REAR_WIPER/1(INIT)
  [INIT] -> FRONT_WIPER/1(INIT)
  [INIT] -> EXTERNAL_LIGHTS/1(INIT)
  [INIT] -> WASHERS/1(INIT)
  [INIT] -> PASSING_AND_HIGH_BEAM/1(INIT)
  [INIT] -> FOG_LAMP/1(INIT)
  PASSING_AND_HIGH_BEAM/2(R_PASSING) -> R_PASSING/1
  PASSING_AND_HIGH_BEAM/1(R_HIGH_BEAM) -> R_HIGH_BEAM/1
  [CSW_LINE_1] -> PASSING_AND_HIGH_BEAM/2(CSW_LINE_1)
  [VEHICLE_STATE] -> EXTERNAL_LIGHTS/4(VEHICLE_STATE)
  [VEHICLE_STATE] -> FRONT_WIPER/4(VEHICLE_STATE)
  VEHICLE_STATE/1 -> [VEHICLE_STATE]
  REAR_WIPER/1(R_RR_WIPER) -> R_RR_WIPER/1
  [CSW_LINE_5] -> REAR_WIPER/2(CSW_LINE_5)
  [CSW_LINE_2] -> INTERMITTENT_TIME/2(CSW_LINE_2)
  [CSW_LINE_5] -> INTERMITTENT_TIME/1(CSW_LINE_5)
  FRONT_WIPER/1(R_FRONT_WIPER) -> R_FRONT_WIPER/1
  [CSW_LINE_6] -> FRONT_WIPER/3(CSW_LINE_6)
  [CSW_LINE_4] -> FRONT_WIPER/2(CSW_LINE_4)
  EXTERNAL_LIGHTS/1(R_EXT_LIGHTS) -> R_EXT_LIGHTS/1
  [CSW_LINE_4] -> EXTERNAL_LIGHTS/3(CSW_LINE_4)
  [CSW_LINE_2] -> EXTERNAL_LIGHTS/2(CSW_LINE_2)
  FLASHERS/1(R_FLASH_LEFT) -> R_FLASH_LEFT/1
  FLASHERS/2(R_FLASH_RIGHT) -> R_FLASH_RIGHT/1
  [CSW_LINE_3] -> FLASHERS/1(CSW_LINE_3)
  CSW_LINE_6/1 -> [CSW_LINE_6]
  CSW_LINE_5/1 -> [CSW_LINE_5]
  CSW_LINE_4/1 -> [CSW_LINE_4]
  CSW_LINE_3/1 -> [CSW_LINE_3]
  CSW_LINE_2/1 -> [CSW_LINE_2]
  WASHERS/1(R_FR_WASHER) -> R_FR_WASHER/1
  WASHERS/2(R_RR_WASHER) -> R_RR_WASHER/1
  [CSW_LINE_3] -> WASHERS/2(CSW_LINE_3)
  FOG_LAMP/2(R_RR_FOG) -> R_RR_FOG/1
  FOG_LAMP/1(R_FR_FOG) -> R_FR_FOG/1
  [CSW_LINE_1] -> FOG_LAMP/2(CSW_LINE_1)
  CSW_LINE_1/1 -> [CSW_LINE_1]
  LIGHTING_CSW_CONFIGURATION_CF/1 -> [LIGHTING_CSW_CONFIGURATION_CF]
  [LIGHTING_CSW_CONFIGURATION_CF] -> EXTERNAL_LIGHTS/5(LIGHTING_CSW_CONFIGURATION_CF)
  DELAY_AFTER_RESET_TM/1 -> [DELAY_AFTER_RESET_TM]
  Constant3/1 -> UnitDelay2/1
  UnitDelay2/1 -> RSA_Timer/1, RSA_SRFlipFlop_v01_02/1
  RSA_DetectIncrease_v01_04/1 -> RSA_SRFlipFlop_v01_02/2
  RSA_SRFlipFlop_v01_02/1 -> [INIT]
  RSA_Timer/1 -> RSA_DetectIncrease_v01_04/1
  RSA_Timer/2 -> Terminator/1
  [DELAY_AFTER_RESET_TM] -> RSA_Timer/2

== system BCM_C1A_CombiSwitch_9/CombiSwitch/CSW_FAILURE_DETECTION ==
  VEHICLE_STATE : Inport  OutDataTypeStr=Enum: TYP_VEHICLE_STATE
      settings: AttributesFormatString=Type : %<OutDataTypeStr>
  RAZ_BY_DIAG : Inport  Port=2  OutDataTypeStr=boolean
      settings: AttributesFormatString=Type : %<OutDataTypeStr>
  CSW_LINE_1 : Inport  Port=3  OutDataTypeStr=boolean  PortDimensions=6
      settings: AttributesFormatString=Type : %<OutDataTypeStr>
  CSW_LINE_2 : Inport  Port=4  OutDataTypeStr=boolean  PortDimensions=6
      settings: AttributesFormatString=Type : %<OutDataTypeStr>
  CSW_LINE_3 : Inport  Port=5  OutDataTypeStr=boolean  PortDimensions=6
      settings: AttributesFormatString=Type : %<OutDataTypeStr>
  CSW_LINE_4 : Inport  Port=6  OutDataTypeStr=boolean  PortDimensions=6
      settings: AttributesFormatString=Type : %<OutDataTypeStr>
  CSW_LINE_5 : Inport  Port=7  OutDataTypeStr=boolean  PortDimensions=6
      settings: AttributesFormatString=Type : %<OutDataTypeStr>
  CSW_LINE_6 : Inport  Port=8  OutDataTypeStr=boolean  PortDimensions=6
      settings: AttributesFormatString=Type : %<OutDataTypeStr>
  COMBI_SW_FAILURE_DETECTED_TM : Inport  Port=9  OutDataTypeStr=uint16
      settings: AttributesFormatString=Type : %<OutDataTypeStr>
  IN_DRIVING_CYCLE : Inport  Port=10  OutDataTypeStr=boolean
      settings: AttributesFormatString=Type : %<OutDataTypeStr>
  CSW_FAILURE_DETECTION_FCT : Stateflow chart  Description=RQT_BCM_CSV_1_0_1  TreatAsAtomicUnit=on
  DET_CSW_FAILURE : Subsystem
  COMBI_SW_FAILURE_TFAIL : Outport  OutDataTypeStr=boolean
      settings: AttributesFormatString=Type : %<OutDataTypeStr>\nInit :%<InitialOutput>
  COMBI_SW_FAILURE_TCONF : Outport  Port=2  OutDataTypeStr=boolean
      settings: AttributesFormatString=Type : %<OutDataTypeStr>\nInit :%<InitialOutput>
  CSW_IN_FAILURE_MODE : Outport  Port=3  OutDataTypeStr=boolean
      settings: AttributesFormatString=Type : %<OutDataTypeStr>\nInit :%<InitialOutput>
  wires:
  IN_DRIVING_CYCLE/1 -> [IN_DRIVING_CYCLE]
  CSW_FAILURE_DETECTION_FCT/2(COMBI_SW_FAILURE_TCONF) -> COMBI_SW_FAILURE_TCONF/1
  [COMBI_SW_FAILURE_DETECTED_TM] -> CSW_FAILURE_DETECTION_FCT/4(COMBI_SW_FAILURE_DETECTED_TM)
  [RAZ_BY_DIAG] -> CSW_FAILURE_DETECTION_FCT/2(RAZ_BY_DIAG)
  [IN_DRIVING_CYCLE] -> CSW_FAILURE_DETECTION_FCT/1(IN_DRIVING_CYCLE)
  [COMBI_SW_FAILURE] -> CSW_FAILURE_DETECTION_FCT/3(COMBI_SW_FAILURE)
  COMBI_SW_FAILURE_DETECTED_TM/1 -> [COMBI_SW_FAILURE_DETECTED_TM]
  [CSW_LINE_6] -> DET_CSW_FAILURE/8(CSW_LINE_6)
  [CSW_LINE_5] -> DET_CSW_FAILURE/7(CSW_LINE_5)
  [CSW_LINE_4] -> DET_CSW_FAILURE/6(CSW_LINE_4)
  [CSW_LINE_3] -> DET_CSW_FAILURE/5(CSW_LINE_3)
  [CSW_LINE_2] -> DET_CSW_FAILURE/4(CSW_LINE_2)
  [CSW_LINE_1] -> DET_CSW_FAILURE/3(CSW_LINE_1)
  [RAZ_BY_DIAG] -> DET_CSW_FAILURE/2(RAZ_BY_DIAG)
  [VEHICLE_STATE] -> DET_CSW_FAILURE/1(VEHICLE_STATE)
  CSW_LINE_6/1 -> [CSW_LINE_6]
  CSW_LINE_5/1 -> [CSW_LINE_5]
  CSW_LINE_4/1 -> [CSW_LINE_4]
  CSW_LINE_3/1 -> [CSW_LINE_3]
  CSW_LINE_2/1 -> [CSW_LINE_2]
  CSW_LINE_1/1 -> [CSW_LINE_1]
  RAZ_BY_DIAG/1 -> [RAZ_BY_DIAG]
  VEHICLE_STATE/1 -> [VEHICLE_STATE]
  CSW_FAILURE_DETECTION_FCT/3(CSW_IN_FAILURE_MODE) -> CSW_IN_FAILURE_MODE/1
  CSW_FAILURE_DETECTION_FCT/1(COMBI_SW_FAILURE_TFAIL) -> COMBI_SW_FAILURE_TFAIL/1
  DET_CSW_FAILURE/1(COMBI_SW_FAILURE) -> [COMBI_SW_FAILURE]

== system BCM_C1A_CombiSwitch_9/CombiSwitch/DET_AUTOMATED_FCT_AVAILABLE ==
  CAR_SECURE_S : Inport  OutDataTypeStr=boolean
      settings: AttributesFormatString=Type : %<OutDataTypeStr>
  DRIVER_DOOR_OPENED : Inport  Port=2  OutDataTypeStr=boolean
      settings: AttributesFormatString=Type : %<OutDataTypeStr>
  SPEED_UNAVAILABLE_OR_INVALID : Inport  Port=3  OutDataTypeStr=boolean
      settings: AttributesFormatString=Type : %<OutDataTypeStr>
  VEHICLE_RUNNING : Inport  Port=4  OutDataTypeStr=boolean
      settings: AttributesFormatString=Type : %<OutDataTypeStr>
  VEHICLE_STATE : Inport  Port=5  OutDataTypeStr=Enum: TYP_VEHICLE_STATE
      settings: AttributesFormatString=Type : %<OutDataTypeStr>
  Constant : Constant  Value=TYP_VEHICLE_STATE.VS_ENGINE_RUNNING  OutDataTypeStr=Enum: TYP_VEHICLE_STATE  SampleTime=-1
  Constant1 : Constant  Value=TYP_VEHICLE_STATE.VS_AUTOACC_LEVEL  OutDataTypeStr=Enum: TYP_VEHICLE_STATE  SampleTime=-1
  Constant3 : Constant  Value=TYP_VEHICLE_STATE.VS_AUTOACC_LEVEL  OutDataTypeStr=Enum: TYP_VEHICLE_STATE  SampleTime=-1
  Constant5 : Constant  Value=TYP_VEHICLE_STATE.VS_AUTOACC_LEVEL  OutDataTypeStr=Enum: TYP_VEHICLE_STATE  SampleTime=-1
  LogicalOperator10 : Logic  Inputs=3  OutDataTypeStr=boolean
  LogicalOperator12 : Logic  Operator=OR  Inputs=3  OutDataTypeStr=boolean
  LogicalOperator14 : Logic  OutDataTypeStr=boolean
  LogicalOperator15 : Logic  Operator=OR  OutDataTypeStr=boolean
  LogicalOperator2 : Logic  Inputs=3  OutDataTypeStr=boolean
  LogicalOperator4 : Logic  Operator=OR  OutDataTypeStr=boolean
  LogicalOperator5 : Logic  Operator=NOT  Inputs=1  OutDataTypeStr=boolean
  LogicalOperator6 : Logic  Operator=NOT  Inputs=1  OutDataTypeStr=boolean
  LogicalOperator9 : Logic  Operator=OR  OutDataTypeStr=boolean
  RSA_DetectIncrease_v01_04 : Renault_Library/Complex blocks/Logic & Bit Operations/RSA_DetectIncrease_v01_04  Tag=[LIB]  chkini=on  vinit=false
      settings: AttributesFormatString=%<MaskType> : Ver : 01.04\nCompare the Input with Initial Value = %<chkini>\nInitial Value : = %<vinit>
  RSA_DetectIncrease_v01_{1,3..6} (5 alike) : Renault_Library/Complex blocks/Logic & Bit Operations/RSA_DetectIncrease_v01_04  Tag=[LIB]  chkini=on  vinit=false
      settings: AttributesFormatString=%<MaskType> : Ver : 01.04\nCompare the Input with Initial Value = %<chkini>\nInitial Value : = %<vinit>
  RSA_SRFlipFlopSetPrioritary_v01_03 : Renault_Library/Complex blocks/Flip-Flop/RSA_SRFlipFlopSetPrioritary_v01_03  Tag=[LIB]  init=false
      settings: AttributesFormatString=%<MaskType> : Ver : 01.03\n<init=%<init>>
  RelationalOperator : RelationalOperator  Operator===  OutDataTypeStr=boolean  RndMeth=Nearest  InputSameDT=on
  RelationalOperator1 : RelationalOperator  Operator=<=  OutDataTypeStr=boolean  RndMeth=Nearest  InputSameDT=on
  RelationalOperator3 : RelationalOperator  Operator=<=  OutDataTypeStr=boolean  RndMeth=Nearest  InputSameDT=on
  RelationalOperator5 : RelationalOperator  Operator=<=  OutDataTypeStr=boolean  RndMeth=Nearest  InputSameDT=on
  IN_DRIVING_CYCLE : Outport  OutDataTypeStr=boolean
      settings: AttributesFormatString=Type : %<OutDataTypeStr>\nInit :%<InitialOutput>
  wires:
  RSA_DetectIncrease_v01_4/1 -> LogicalOperator12/2
  RSA_DetectIncrease_v01_3/1 -> LogicalOperator12/1
  RSA_DetectIncrease_v01_6/1 -> LogicalOperator15/2
  RSA_DetectIncrease_v01_5/1 -> LogicalOperator12/3
  LogicalOperator12/1 -> LogicalOperator14/2
  RelationalOperator5/1 -> LogicalOperator14/1
  LogicalOperator14/1 -> LogicalOperator15/1
  Constant5/1 -> RelationalOperator5/2
  [VEHICLE_STATE] -> RelationalOperator5/1
  [CAR_SECURE_S] -> RSA_DetectIncrease_v01_4/1
  [DRIVER_DOOR_OPENED] -> RSA_DetectIncrease_v01_5/1
  [SPEED_UNAVAILABLE_OR_INVALID] -> RSA_DetectIncrease_v01_3/1
  [DRIVER_DOOR_OPENED] -> LogicalOperator9/2
  [CAR_SECURE_S] -> LogicalOperator9/1
  CAR_SECURE_S/1 -> [CAR_SECURE_S]
  DRIVER_DOOR_OPENED/1 -> [DRIVER_DOOR_OPENED]
  LogicalOperator10/1 -> LogicalOperator4/2
  LogicalOperator15/1 -> LogicalOperator10/1
  [SPEED_UNAVAILABLE_OR_INVALID] -> LogicalOperator10/2
  LogicalOperator4/1 -> RSA_SRFlipFlopSetPrioritary_v01_03/2
  RelationalOperator3/1 -> RSA_DetectIncrease_v01_6/1
  Constant3/1 -> RelationalOperator3/2
  [VEHICLE_STATE] -> RelationalOperator3/1
  LogicalOperator6/1 -> LogicalOperator2/3
  LogicalOperator5/1 -> LogicalOperator2/2
  LogicalOperator2/1 -> LogicalOperator4/1
  [SPEED_UNAVAILABLE_OR_INVALID] -> LogicalOperator6/1
  [VEHICLE_RUNNING] -> LogicalOperator5/1
  RSA_DetectIncrease_v01_1/1 -> LogicalOperator2/1
  VEHICLE_RUNNING/1 -> [VEHICLE_RUNNING]
  SPEED_UNAVAILABLE_OR_INVALID/1 -> [SPEED_UNAVAILABLE_OR_INVALID]
  RelationalOperator1/1 -> RSA_DetectIncrease_v01_1/1
  Constant1/1 -> RelationalOperator1/2
  [VEHICLE_STATE] -> RelationalOperator1/1
  RelationalOperator/1 -> RSA_DetectIncrease_v01_04/1
  RSA_DetectIncrease_v01_04/1 -> RSA_SRFlipFlopSetPrioritary_v01_03/1
  Constant/1 -> RelationalOperator/2
  [VEHICLE_STATE] -> RelationalOperator/1
  VEHICLE_STATE/1 -> [VEHICLE_STATE]
  RSA_SRFlipFlopSetPrioritary_v01_03/1 -> IN_DRIVING_CYCLE/1
  LogicalOperator9/1 -> LogicalOperator10/3

== system BCM_C1A_CombiSwitch_9/CombiSwitch/LIGHTING_FAILURE_DETECTION ==
  VEHICLE_STATE : Inport  OutDataTypeStr=Enum: TYP_VEHICLE_STATE
      settings: AttributesFormatString=Type : %<OutDataTypeStr>
  RAZ_BY_DIAG : Inport  Port=2  OutDataTypeStr=boolean
      settings: AttributesFormatString=Type : %<OutDataTypeStr>
  CSW_LINE_2 : Inport  Port=3  OutDataTypeStr=boolean  PortDimensions=6
      settings: AttributesFormatString=Type : %<OutDataTypeStr>
  CSW_LINE_4 : Inport  Port=4  OutDataTypeStr=boolean  PortDimensions=6
      settings: AttributesFormatString=Type : %<OutDataTypeStr>
  IN_DRIVING_CYCLE : Inport  Port=5  OutDataTypeStr=boolean
      settings: AttributesFormatString=Type : %<OutDataTypeStr>
  COMBI_SW_FAILURE_DETECTED_TM : Inport  Port=6  OutDataTypeStr=uint16
      settings: AttributesFormatString=Type : %<OutDataTypeStr>
  LIGHTING_CSW_CONFIGURATION_CF : Inport  Port=7  OutDataTypeStr=Enum: TYP_LIGHTING_CSW
      settings: AttributesFormatString=Type : %<OutDataTypeStr>
  Constant : Constant  Value=TYP_LIGHTING_CSW.LIGHTING_CSW_FOR_EUROPE  OutDataTypeStr=Enum: TYP_LIGHTING_CSW  SampleTime=-1
  Constant1 : Constant  Value=TYP_LIGHTING_CSW.LIGHTING_CSW_WORLD_WITHOUT_ALS  OutDataTypeStr=Enum: TYP_LIGHTING_CSW  SampleTime=-1
  Constant2 : Constant  Value=TYP_LIGHTING_CSW.LIGHTING_CSW_WORLD_WITH_ALS  OutDataTypeStr=Enum: TYP_LIGHTING_CSW  SampleTime=-1
  DET_LIGHTING_FAILURE_3_POSITIONS : Subsystem  Description=|  TreatAsAtomicUnit=on
      | RQT_BCM_CSV_1_8
      | RQT_BCM_CSV_1_8_0
      settings: RTWSystemCode=Inline
  DET_LIGHTING_FAILURE_4_POSITIONS : Subsystem  Description=RQT_BCM_CSV_1_8_1  TreatAsAtomicUnit=on
      settings: RTWSystemCode=Inline
  LIGHTING_FAILURE_DETECTION_FCT : Stateflow chart  Description=|  TreatAsAtomicUnit=on
      | RQT_BCM_CSV_1_8_0
      | RQT_BCM_CSV_1_8_1
      | RQT_BCM_CSV_1_8
  LogicalOperator : Logic  Operator=OR  OutDataTypeStr=boolean
  LogicalOperator1 : Logic  Operator=OR  OutDataTypeStr=boolean
  RelationalOperator : RelationalOperator  Operator===  OutDataTypeStr=boolean  RndMeth=Nearest  InputSameDT=on
  RelationalOperator1 : RelationalOperator  Operator===  OutDataTypeStr=boolean  RndMeth=Nearest  InputSameDT=on
  RelationalOperator2 : RelationalOperator  Operator===  OutDataTypeStr=boolean  RndMeth=Nearest  InputSameDT=on
  COMBI_SW_LIGHTING_FAILURE_TFAIL : Outport  OutDataTypeStr=boolean
      settings: AttributesFormatString=Type : %<OutDataTypeStr>\nInit :%<InitialOutput>
  COMBI_SW_LIGHTING_FAILURE_TCONF : Outport  Port=2  OutDataTypeStr=boolean
      settings: AttributesFormatString=Type : %<OutDataTypeStr>\nInit :%<InitialOutput>
  LIGHTING_CSW_FAILURE_MODE : Outport  Port=3  OutDataTypeStr=boolean
      settings: AttributesFormatString=Type : %<OutDataTypeStr>\nInit :%<InitialOutput>
  wires:
  IN_DRIVING_CYCLE/1 -> [IN_DRIVING_CYCLE]
  LIGHTING_FAILURE_DETECTION_FCT/3(LIGHTING_CSW_FAILURE_MODE) -> LIGHTING_CSW_FAILURE_MODE/1
  LIGHTING_FAILURE_DETECTION_FCT/2(COMBI_SW_LIGHTING_FAILURE_TCONF) -> COMBI_SW_LIGHTING_FAILURE_TCONF/1
  LIGHTING_FAILURE_DETECTION_FCT/1(COMBI_SW_LIGHTING_FAILURE_TFAIL) -> COMBI_SW_LIGHTING_FAILURE_TFAIL/1
  [COMBI_SW_FAILURE_DETECTED_TM] -> LIGHTING_FAILURE_DETECTION_FCT/4(COMBI_SW_FAILURE_DETECTED_TM)
  [RAZ_BY_DIAG] -> LIGHTING_FAILURE_DETECTION_FCT/2(RAZ_BY_DIAG)
  [IN_DRIVING_CYCLE] -> LIGHTING_FAILURE_DETECTION_FCT/1(IN_DRIVING_CYCLE)
  [COMBI_SW_LIGHTING_FAILURE] -> LIGHTING_FAILURE_DETECTION_FCT/3(COMBI_SW_LIGHTING_FAILURE)
  COMBI_SW_FAILURE_DETECTED_TM/1 -> [COMBI_SW_FAILURE_DETECTED_TM]
  DET_LIGHTING_FAILURE_4_POSITIONS/1(COMBI_SW_LIGHTING_FAILURE_4_POS) -> LogicalOperator1/1
  [CSW_LINE_4] -> DET_LIGHTING_FAILURE_4_POSITIONS/4(CSW_LINE_4)
  [CSW_LINE_2] -> DET_LIGHTING_FAILURE_4_POSITIONS/3(CSW_LINE_2)
  [RAZ_BY_DIAG] -> DET_LIGHTING_FAILURE_4_POSITIONS/2(RAZ_BY_DIAG)
  [VEHICLE_STATE] -> DET_LIGHTING_FAILURE_4_POSITIONS/1(VEHICLE_STATE)
  CSW_LINE_4/1 -> [CSW_LINE_4]
  CSW_LINE_2/1 -> [CSW_LINE_2]
  RAZ_BY_DIAG/1 -> [RAZ_BY_DIAG]
  VEHICLE_STATE/1 -> [VEHICLE_STATE]
  LIGHTING_CSW_CONFIGURATION_CF/1 -> [LIGHTING_CSW_CONFIGURATION_CF]
  [CSW_LINE_4] -> DET_LIGHTING_FAILURE_3_POSITIONS/4(CSW_LINE_4)
  [CSW_LINE_2] -> DET_LIGHTING_FAILURE_3_POSITIONS/3(CSW_LINE_2)
  [RAZ_BY_DIAG] -> DET_LIGHTING_FAILURE_3_POSITIONS/2(RAZ_BY_DIAG)
  [VEHICLE_STATE] -> DET_LIGHTING_FAILURE_3_POSITIONS/1(VEHICLE_STATE)
  DET_LIGHTING_FAILURE_3_POSITIONS/1(COMBI_SW_LIGHTING_FAILURE_3_POS) -> LogicalOperator1/2
  [LIGHTING_CSW_CONFIGURATION_CF] -> RelationalOperator/1
  [LIGHTING_CSW_CONFIGURATION_CF] -> RelationalOperator1/1
  Constant2/1 -> RelationalOperator1/2
  RelationalOperator1/1 -> DET_LIGHTING_FAILURE_4_POSITIONS/Enable
  Constant/1 -> RelationalOperator/2
  Constant1/1 -> RelationalOperator2/2
  [LIGHTING_CSW_CONFIGURATION_CF] -> RelationalOperator2/1
  RelationalOperator/1 -> LogicalOperator/1
  RelationalOperator2/1 -> LogicalOperator/2
  LogicalOperator/1 -> DET_LIGHTING_FAILURE_3_POSITIONS/Enable
  LogicalOperator1/1 -> [COMBI_SW_LIGHTING_FAILURE]
